simulink model "fm"  (R2024b)
settings: Solver=VariableStepAuto  StartTime=0.0  StopTime=2  MaxStep=0.1  RelTol=1e-3
undefined symbols (not defined in the file): designMultirateFIR, DiscIntNeverNeededParam, dspblkCoreblockFVToolHelper, gcbh
libraries: dspvision x4, dspmlti4 x2
settings Model: Creator=mahir  LastModifiedBy=Asus
settings ModelReferenceCC: EnableRefExpFcnMdlSchedulingChecks=on
settings RTWCC: GPUComputeCapability=3.5

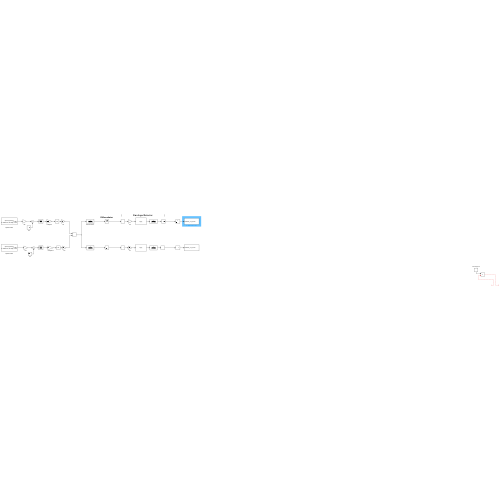
[thumbnail: Simulink's stored preview of the top-level diagram]
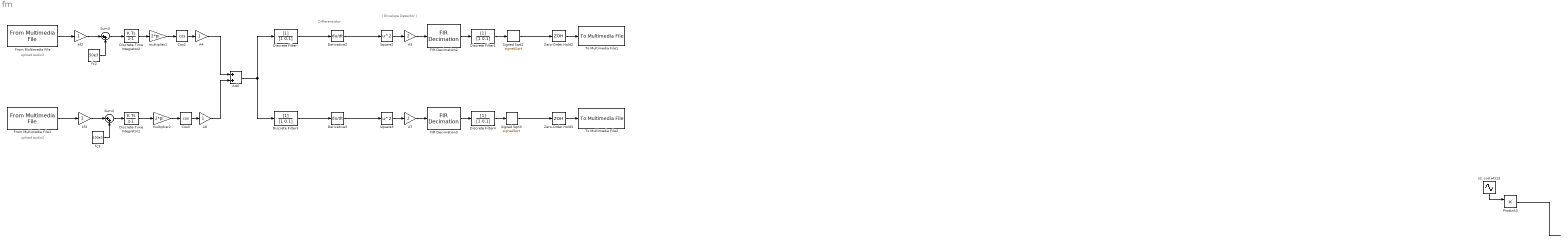
== system fm ==
  note: upload audio3
  note: Differentiator
  note: | Envelope Detector |
  note: upload audio2
  A4 : Gain
  A5 : Gain  Gain=2
  A6 : Gain
  A7 : Gain  Gain=2
  Add : Sum
  Cos2 : Trigonometry  Operator=cos
  Cos3 : Trigonometry  Operator=cos
  Derivative2 : Derivative
  Derivative3 : Derivative
  Discrete Filter- : DiscreteFilter  LoadFcn=dspblkCoreblockFVToolHelper(gcbh,'load');  Denominator=[1 0.1]
      settings: CopyFcn=dspblkCoreblockFVToolHelper(gcbh,'copy');  DeleteFcn=dspblkCoreblockFVToolHelper(gcbh,'close');  ModelCloseFcn=dspblkCoreblockFVToolHelper(gcbh,'close');  PreSaveFcn=dspblkCoreblockFVToolHelper(gcbh,'presave');  PostSaveFcn=dspblkCoreblockFVToolHelper(gcbh,'postsave');  CloseFcn=dspblkCoreblockFVToolHelper(gcbh,'close');
  Discrete Filter1 : DiscreteFilter  LoadFcn=dspblkCoreblockFVToolHelper(gcbh,'load');  Denominator=[1 0.1]
      settings: CopyFcn=dspblkCoreblockFVToolHelper(gcbh,'copy');  DeleteFcn=dspblkCoreblockFVToolHelper(gcbh,'close');  ModelCloseFcn=dspblkCoreblockFVToolHelper(gcbh,'close');  PreSaveFcn=dspblkCoreblockFVToolHelper(gcbh,'presave');  PostSaveFcn=dspblkCoreblockFVToolHelper(gcbh,'postsave');  CloseFcn=dspblkCoreblockFVToolHelper(gcbh,'close');
  Discrete Filter3 : DiscreteFilter  LoadFcn=dspblkCoreblockFVToolHelper(gcbh,'load');  Denominator=[1 0.1]
      settings: CopyFcn=dspblkCoreblockFVToolHelper(gcbh,'copy');  DeleteFcn=dspblkCoreblockFVToolHelper(gcbh,'close');  ModelCloseFcn=dspblkCoreblockFVToolHelper(gcbh,'close');  PreSaveFcn=dspblkCoreblockFVToolHelper(gcbh,'presave');  PostSaveFcn=dspblkCoreblockFVToolHelper(gcbh,'postsave');  CloseFcn=dspblkCoreblockFVToolHelper(gcbh,'close');
  Discrete Filter4 : DiscreteFilter  LoadFcn=dspblkCoreblockFVToolHelper(gcbh,'load');  Denominator=[1 0.1]
      settings: CopyFcn=dspblkCoreblockFVToolHelper(gcbh,'copy');  DeleteFcn=dspblkCoreblockFVToolHelper(gcbh,'close');  ModelCloseFcn=dspblkCoreblockFVToolHelper(gcbh,'close');  PreSaveFcn=dspblkCoreblockFVToolHelper(gcbh,'presave');  PostSaveFcn=dspblkCoreblockFVToolHelper(gcbh,'postsave');  CloseFcn=dspblkCoreblockFVToolHelper(gcbh,'close');
  Discrete-Time Integrator1 : DiscreteIntegrator  SampleTime=-1  ICPrevOutput=DiscIntNeverNeededParam  ICPrevScaledInput=DiscIntNeverNeededParam
  Discrete-Time Integrator2 : DiscreteIntegrator  SampleTime=-1  ICPrevOutput=DiscIntNeverNeededParam  ICPrevScaledInput=DiscIntNeverNeededParam
  FIR Decimation2 : dspmlti4/FIR Decimation  FilterSource=Auto  h=designMultirateFIR(1,2)  D=1  filtStruct=Direct form  FilterObject=FDECIM  InputProcessing=Columns as channels (frame based)  framing=Enforce single-rate processing  AllowArbitraryInputLength=off  inputOffset=0  outputBufInitCond=0  roundingMode=Floor  overflowMode=off  firstCoeffDataTypeStr=Inherit: Same word length as input  firstCoeffMin=[]  firstCoeffMax=[]  firstCoeffLastDataTypeStr=Inherit: Same word length as input  outputDataTypeStr=Inherit: Same as accumulator  outputMin=[]  outputMax=[]  outputLastDataTypeStr=Inherit: Same as accumulator
  FIR Decimation3 : dspmlti4/FIR Decimation  FilterSource=Auto  h=designMultirateFIR(1,2)  D=1  filtStruct=Direct form  FilterObject=FDECIM  InputProcessing=Columns as channels (frame based)  framing=Enforce single-rate processing  AllowArbitraryInputLength=off  inputOffset=0  outputBufInitCond=0  roundingMode=Floor  overflowMode=off  firstCoeffDataTypeStr=Inherit: Same word length as input  firstCoeffMin=[]  firstCoeffMax=[]  firstCoeffLastDataTypeStr=Inherit: Same word length as input  outputDataTypeStr=Inherit: Same as accumulator  outputMin=[]  outputMax=[]  outputLastDataTypeStr=Inherit: Same as accumulator
  From Multimedia File : dspvision/From Multimedia File  inputFilename=speech_dft.mp3  readRange=[1 Inf]  loop=on  numPlays=inf  outputStreams=Audio only  videoDataType=single  audioDataType=double  inheritSampleTime=on  userDefinedSampleTime=1/30  noAudioOutput=off  isIntensityVideo=off  fourcc=RGB  colorVideoFormat=Separate color signals  outputEOF=off  dataOrg=Column-major  audioFrameSize=1024  computeAudioFrameSize=off  outSamplingMode=Sample based
      settings: LibrarySourceBlock=audiosources/From Multimedia File
  From Multimedia File1 : dspvision/From Multimedia File  inputFilename=speech_dft.mp3  readRange=[1 Inf]  loop=on  numPlays=inf  outputStreams=Audio only  videoDataType=single  audioDataType=double  inheritSampleTime=on  userDefinedSampleTime=1/30  noAudioOutput=off  isIntensityVideo=off  fourcc=RGB  colorVideoFormat=Separate color signals  outputEOF=off  dataOrg=Column-major  audioFrameSize=1024  computeAudioFrameSize=off  outSamplingMode=Sample based
      settings: LibrarySourceBlock=audiosources/From Multimedia File
  Product3 : Product
  Signed Sqrt2 : Sqrt  Operator=signedSqrt
  Signed Sqrt3 : Sqrt  Operator=signedSqrt
  Square2 : Math  Operator=square
  Square3 : Math  Operator=square
  Sum3 : Sum  Inputs=|++
  Sum4 : Sum  Inputs=|++
  To Multimedia File1 : dspvision/To Multimedia File  outputFilename=C:\Users\fm_out_2.wav  streamSelection=Audio only  videoCompressor=None (uncompressed)  audioCompressor=None (uncompressed)  imagePorts=One multidimensional signal  fileType=WAV  audioDatatype=16-bit integer  fourcc=RGB  audioBitRate=128  audioQuality=75  videoQuality=75  mj2000CompFactor=10
      settings: LibrarySourceBlock=dspsnks4/To Multimedia File
  To Multimedia File2 : dspvision/To Multimedia File  outputFilename=C:\Users\fm_out_3.wav  streamSelection=Audio only  videoCompressor=None (uncompressed)  audioCompressor=None (uncompressed)  imagePorts=One multidimensional signal  fileType=WAV  audioDatatype=16-bit integer  fourcc=RGB  audioBitRate=128  audioQuality=75  videoQuality=75  mj2000CompFactor=10
      settings: LibrarySourceBlock=dspsnks4/To Multimedia File
  Zero-Order Hold2 : ZeroOrderHold  SampleTime=-1
  Zero-Order Hold3 : ZeroOrderHold  SampleTime=-1
  fc2 : Constant  Value=50e3
  fc3 : Constant  Value=100e3
  kf2 : Gain
  kf3 : Gain
  multiplier1 : Gain  Gain=2*pi
  multiplier2 : Gain  Gain=2*pi
  s2: cos(wt)13 : Sin  Frequency=2*pi*50e3  Phase=-pi/2  SampleTime=1024
  wires:
  fc2/1 -> Sum3/2
  From Multimedia File/1 -> kf2/1
  Sum3/1 -> Discrete-Time Integrator2/1
  Cos2/1 -> A4/1
  Square2/1 -> A5/1
  kf2/1 -> Sum3/1
  multiplier1/1 -> Cos2/1
  Discrete-Time Integrator2/1 -> multiplier1/1
  A5/1 -> FIR Decimation2/1
  Zero-Order Hold2/1 -> To Multimedia File1/1
  Discrete Filter4/1 -> Signed Sqrt3/1
  Zero-Order Hold3/1 -> To Multimedia File2/1
  FIR Decimation3/1 -> Discrete Filter4/1
  Sum4/1 -> Discrete-Time Integrator1/1
  A7/1 -> FIR Decimation3/1
  Signed Sqrt3/1 -> Zero-Order Hold3/1
  multiplier2/1 -> Cos3/1
  Cos3/1 -> A6/1
  From Multimedia File1/1 -> kf3/1
  Discrete-Time Integrator1/1 -> multiplier2/1
  kf3/1 -> Sum4/1
  fc3/1 -> Sum4/2
  Square3/1 -> A7/1
  FIR Decimation2/1 -> Discrete Filter1/1
  Derivative3/1 -> Square3/1
  ? -> Product3/2
  Product3/1 -> ?
  s2: cos(wt)13/1 -> Product3/1
  Signed Sqrt2/1 -> Zero-Order Hold2/1
  Derivative2/1 -> Square2/1
  Discrete Filter1/1 -> Signed Sqrt2/1
  A6/1 -> Add/2
  A4/1 -> Add/1
  Add/1 -> Discrete Filter-/1, Discrete Filter3/1
  Discrete Filter-/1 -> Derivative2/1
  Discrete Filter3/1 -> Derivative3/1
